simulink model "svpwmDCM"  (R2022b)
settings: Solver=VariableStepAuto  StartTime=0.0  StopTime=0.3  FixedStep=1e-5  RelTol=1e-4  EnableMultiTasking=on
libraries: spsIGBTDiodeLib x12, spsDiodeLib x6, spsSeriesRLCBranchLib x3, spsDCVoltageSourceLib x2, spsGroundLib x2, spsThreePhaseVIMeasurementLib x2, spsPermanentMagnetSynchronousMachineLib x1, spsAlphaBetaZerotodq0Lib x1, simulink x1, spsVoltageMeasurementLib x1, sps_lib x1
settings Model: Creator=Ranit  LastModifiedBy=ahmetcan.akuz
settings SolverCC: AlgebraicLoopSolver=TrustRegion
settings DataIOCC: ReturnWorkspaceOutputs=off
settings OptimizationCC: LifeSpan=inf
settings DebuggingCC: UnconnectedInputMsg=warning  UnconnectedOutputMsg=warning  UnconnectedLineMsg=warning  SFUnexpectedBacktrackingDiag=warning  SFNoUnconditionalDefaultTransitionDiag=warning  SFMachineParentedDataDiag=warning  ArithmeticOperatorsInVariantConditions=warning
settings ModelReferenceCC: EnableRefExpFcnMdlSchedulingChecks=on
settings SFSimCC: SimUseLocalCustomCode=off  CustomCodeUndefinedFunction=UseInterfaceOnly
settings RTWCC: RTWUseLocalCustomCode=off
settings CodeAppCC: StateflowObjectComments=on
settings GRTTargetCC: TargetLangStandard=C89/C90 (ANSI)
settings ConfigComp: CovMetricSettings=dw  CovSaveCumulativeToWorkspaceVar=on  CovSaveSingleToWorkspaceVar=on  CovExternalEMLEnable=off
settings SimscapeCC: SimscapeNormalizeSystem=off

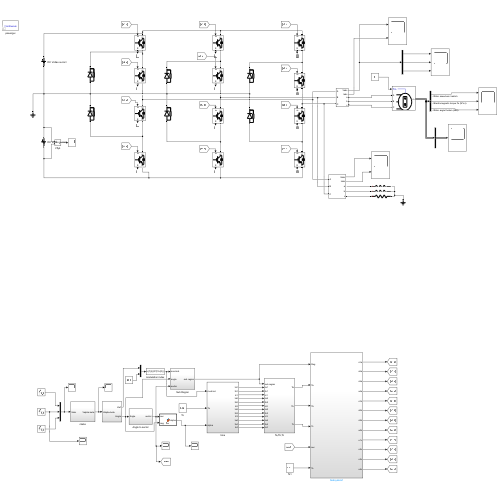
[thumbnail: Simulink's stored preview of the top-level diagram]
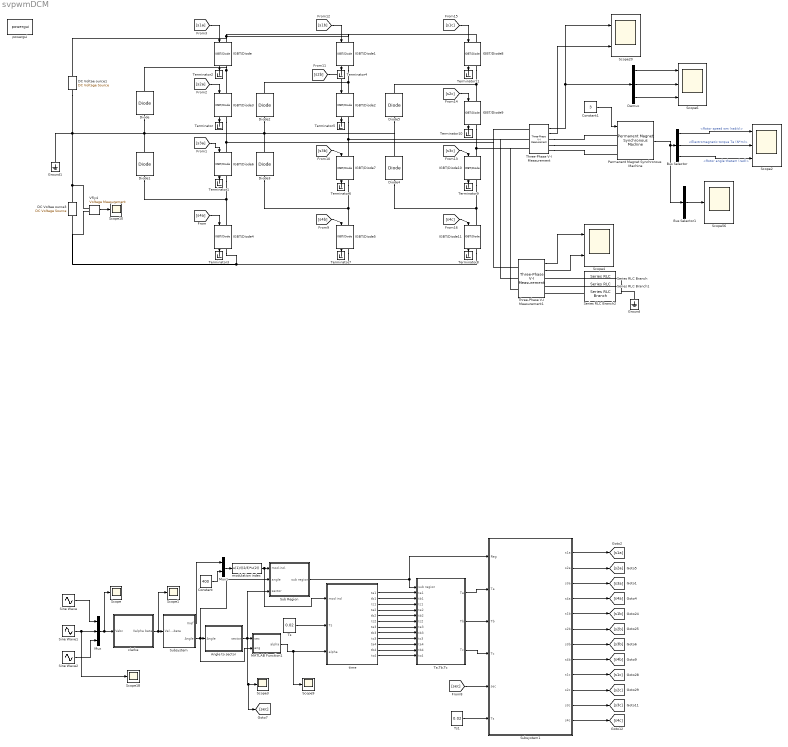
== system svpwmDCM ==
  Angle to sector : Subsystem
  Bus Selector : BusSelector  OutputSignals=Rotor speed wm (rad/s),Electromagnetic torque Te (N*m),Rotor angle thetam (rad)
  Bus Selector1 : BusSelector  OutputSignals=Stator current is_a (A),Stator current is_b (A),Stator current is_c (A)  OutputAsBus=on
  Constant : Constant  Value=400
  Constant1 : Constant  Value=3
  DC Voltae ource1 : spsDCVoltageSourceLib/DC Voltage Source  Amplitude=200  Measurements=None
  DC Voltae ource3 : spsDCVoltageSourceLib/DC Voltage Source  Amplitude=200  Measurements=None
  Demux : Demux  Outputs=3
  Diode{,1..5} (6 alike) : spsDiodeLib/Diode  Ron=0.001  Lon=0  Vf=0.8  IC=0  UseSnubber=off  Rs=500  Cs=250e-9  Measurements=off
  Ground : spsGroundLib/Ground  LConnTagsString=a
  Ground1 : spsGroundLib/Ground  LConnTagsString=a
  IGBT/Diode{,1..11} (12 alike) : spsIGBTDiodeLib/IGBT//Diode  Ron=1e-3  Rs=1e5  Cs=inf  Measurements=on
  MATLAB Function1 : MATLAB Function  TreatAsAtomicUnit=on
  Mux : Mux  Inputs=3
  Mux1 : Mux  Inputs=2
  Permanent Magnet Synchronous Machine : spsPermanentMagnetSynchronousMachineLib/Permanent Magnet Synchronous Machine  NbPhases=3  FluxDistribution=Sinusoidal  RotorType=Round  MechanicalLoad=Torque Tm  PresetModel=No  ShowDetailedParameters=on  MeasurementBus=off  Resistance=12.8  Inductance=8.5e-3  dqInductances=[0.002547 0.002816]  La=0.002682  MachineConstant=Flux linkage established by magnets (V.s)  Flux=0.22  VoltageCst=79.8072  TorqueCst=0.66  Flat=120  Mechanical=[2.26e-05 1.349e-05 2 0]  PolePairs=2  InitialConditions=[0,0, 0,0]  InitialConditions5ph=[0 0 0 0 0 0]  RefAngle=90 degrees behind phase A axis (modified Park)  IterativeDiscreteModel=Trapezoidal non iterative  TsBlock=-1  TsPowergui=0
  Scope{,1,3,9..10,18,56} (7 alike) : Scope
  Scope2 : Scope  NumInputPorts=3
  Scope20 : Scope  NumInputPorts=2
  Scope4 : Scope  NumInputPorts=2
  Scope6 : Scope  NumInputPorts=3
  Series RLC Branch : spsSeriesRLCBranchLib/Series RLC Branch  LConnTagsString=__new0  RConnTagsString=__new0  BranchType=R  Resistance=5  Inductance=20e-6  SetiL0=off  InitialCurrent=0  Capacitance=1e-6  Setx0=off  InitialVoltage=0  Measurements=None
  Series RLC Branch1 : spsSeriesRLCBranchLib/Series RLC Branch  LConnTagsString=__new0  RConnTagsString=__new0  BranchType=R  Resistance=5  Inductance=20e-6  SetiL0=off  InitialCurrent=0  Capacitance=1e-6  Setx0=off  InitialVoltage=0  Measurements=None
  Series RLC Branch2 : spsSeriesRLCBranchLib/Series RLC Branch  LConnTagsString=__new0  RConnTagsString=__new0  BranchType=R  Resistance=5  Inductance=20e-6  SetiL0=off  InitialCurrent=0  Capacitance=1e-6  Setx0=off  InitialVoltage=0  Measurements=None
  Sine Wave : Sin  Amplitude=230  Frequency=2*pi*50  SampleTime=0
  Sine Wave1 : Sin  Amplitude=230  Frequency=2*pi*50  Phase=4*pi/3  SampleTime=0
  Sine Wave2 : Sin  Amplitude=230  Frequency=2*pi*50  Phase=2*pi/3  SampleTime=0
  Sub Region : Subsystem
  Subsystem : Subsystem
  Subsystem1 : Subsystem
  Ta,Tb,Tc : Subsystem
  Terminator{,1..11} (12 alike) : Terminator
  Three-Phase V-I Measurement : spsThreePhaseVIMeasurementLib/Three-Phase V-I Measurement  VoltageMeasurement=phase-to-phase  SetLabelV=off  LabelV=Vabc  Vpu=off  VpuLL=off  CurrentMeasurement=yes  SetLabelI=off  LabelI=Iabc  Ipu=off  Pbase=100e6  Vbase=500e3  OutputType=Complex  PhasorSimulation=off  PSBequivalent=0
  Three-Phase V-I Measurement1 : spsThreePhaseVIMeasurementLib/Three-Phase V-I Measurement  VoltageMeasurement=phase-to-ground  SetLabelV=off  LabelV=Vabc  Vpu=off  VpuLL=off  CurrentMeasurement=yes  SetLabelI=off  LabelI=Iabc  Ipu=off  Pbase=100e6  Vbase=500e3  OutputType=Complex  PhasorSimulation=off  PSBequivalent=0
  Ts : Constant  Value=0.02
  Ts1 : Constant  Value=0.02
  Vfly4 : spsVoltageMeasurementLib/Voltage Measurement  PhasorSimulation=off  OutputType=Complex  PSBequivalent=0
  clarke : Subsystem
  modulation index : Fcn  Expr=u(1)/((2/3)*u(2))
  powergui : sps_lib/powergui  Priority=1  SimulationMode=Continuous  SampleTime=5e-4  frequency=60  Iterations=50  frequencyindice=0  Pbase=100e6  ErrMax=1e-4  UnitsV=kV  UnitsW=MW  buscounter=0  FunctionMessages=off  echomessages=off  EnableUseOfTLC=off  CurrentSourceSwitches=on  DisableSnubberDevices=off  DisableRonSwitches=off  DisableVfSwitches=off  DisplayEquations=off  AutomaticDiscreteSolvers=off  SolverType=Tustin/Backward Euler (TBE)  Interpol=off  ExternalGateDelay=off  methode=off  Ts=10  x0status=blocks  SPID=off  SwTol=0  HookPort=off  NonlinearTolerance=1e-4  nMaxIteration=100  ContinueOnMaxIteration=off  RestoreLinks=warning  ResistiveCurrentMeasurement=off  Frange=[0:2:500]  Ylog=off  Xlog=on  ShowGrid=off  save=off  variable=ZData  structure=ScopeData2  ZoomFFT=off  StartTime=0.0  cycles=1  DisplayStyle=1  fundamental=50  FreqAxis=off  MaxFrequency=1000  frequencyindicesteady=1  RmsSteady=1  display=off
  time : Subsystem
  wires:
  Sine Wave/1 -> Mux/1
  Sine Wave1/1 -> Scope18/1, Mux/2
  Sine Wave2/1 -> Mux/3
  Mux/1 -> clarke/1(Vabc), Scope/1
  clarke/1(Valpha beta) -> Scope1/1, Subsystem/1(Valpha-beta)
  Subsystem/1(Vref) -> Mux1/1
  Constant/1 -> Mux1/2
  Mux1/1 -> modulation index/1
  [s4a] -> IGBT/Diode4/1
  [s3a] -> IGBT/Diode6/1
  [s1a] -> IGBT/Diode/1
  [s2a] -> IGBT/Diode3/1
  Ts/1 -> time/2(Ts)
  time/1(ta1) -> Ta,Tb,Tc/2(ta1)
  time/2(tb1) -> Ta,Tb,Tc/3(tb1)
  time/3(tc1) -> Ta,Tb,Tc/4(tc1)
  time/4(ta2) -> Ta,Tb,Tc/5(ta2)
  time/5(tb2) -> Ta,Tb,Tc/6(tb2)
  time/6(tc2) -> Ta,Tb,Tc/7(tc2)
  time/7(ta3) -> Ta,Tb,Tc/8(ta3)
  time/9(tc3) -> Ta,Tb,Tc/10(tc3)
  time/10(ta4) -> Ta,Tb,Tc/11(ta4)
  time/11(tb4) -> Ta,Tb,Tc/12(tb4)
  time/12(tc4) -> Ta,Tb,Tc/13(tc4)
  time/8(tb3) -> Ta,Tb,Tc/9(tb3)
  modulation index/1 -> time/1(mod ind), Sub Region/1(mod.ind.)
  Subsystem/2(Angle) -> MATLAB Function1/2(ang), Sub Region/2(angle), Angle to sector/1(Angle)
  MATLAB Function1/1(alpha) -> Scope9/1, time/3(alpha)
  [s4b] -> IGBT/Diode5/1
  [s3b] -> IGBT/Diode7/1
  [s1b] -> IGBT/Diode1/1
  [s2b] -> IGBT/Diode2/1
  [s4c] -> IGBT/Diode11/1
  [s3c] -> IGBT/Diode10/1
  [s1c] -> IGBT/Diode8/1
  [s2c] -> IGBT/Diode9/1
  Vfly4/1 -> Scope10/1
  Sub Region/1(sub region) -> Subsystem1/1(Reg), Ta,Tb,Tc/1(sub region)
  Angle to sector/1(sector) -> Sub Region/3(sector), [sec], Scope3/1, MATLAB Function1/1(sec)
  Ta,Tb,Tc/1(Ta) -> Subsystem1/2(Ta)
  Ta,Tb,Tc/2(Tb) -> Subsystem1/3(Tb)
  Ta,Tb,Tc/3(Tc) -> Subsystem1/4(Tc)
  Subsystem1/1(s1a) -> [s1a]
  Subsystem1/2(s2a) -> [s2a]
  Subsystem1/3(s3a) -> [s3a]
  Subsystem1/4(s4a) -> [s4a]
  Subsystem1/6(s2b) -> [s2b]
  Subsystem1/5(s1b) -> [s1b]
  Subsystem1/7(s3b) -> [s3b]
  Subsystem1/8(s4b) -> [s4b]
  Subsystem1/9(s1c) -> [s1c]
  Subsystem1/10(s2c) -> [s2c]
  Subsystem1/11(s3c) -> [s3c]
  Subsystem1/12(s4c) -> [s4c]
  [sec] -> Subsystem1/5(sec)
  Ts1/1 -> Subsystem1/6(Ts)
  Permanent Magnet Synchronous Machine/1 -> Bus Selector1/1, Bus Selector/1
  Constant1/1 -> Permanent Magnet Synchronous Machine/1
  Bus Selector/1 -> Scope2/1  "<Rotor speed wm (rad/s)>"
  Bus Selector/2 -> Scope2/2  "<Electromagnetic torque Te (N*m)>"
  Bus Selector/3 -> Scope2/3  "<Rotor angle thetam (rad)>"
  Bus Selector1/1 -> Scope56/1
  IGBT/Diode3/1 -> Terminator/1
  IGBT/Diode6/1 -> Terminator1/1
  IGBT/Diode/1 -> Terminator2/1
  IGBT/Diode4/1 -> Terminator3/1
  IGBT/Diode1/1 -> Terminator4/1
  IGBT/Diode2/1 -> Terminator5/1
  IGBT/Diode7/1 -> Terminator6/1
  IGBT/Diode5/1 -> Terminator7/1
  IGBT/Diode11/1 -> Terminator8/1
  IGBT/Diode10/1 -> Terminator9/1
  IGBT/Diode9/1 -> Terminator10/1
  IGBT/Diode8/1 -> Terminator11/1
  Three-Phase V-I Measurement/2 -> Scope20/2
  Three-Phase V-I Measurement1/1 -> Scope4/1
  Three-Phase V-I Measurement1/2 -> Scope4/2
  Demux/1 -> Scope6/1
  Demux/2 -> Scope6/2
  Demux/3 -> Scope6/3
  Three-Phase V-I Measurement/1 -> Demux/1, Scope20/1
  connections:
  Diode1/LConn1 -- IGBT/Diode4/LConn1 -- IGBT/Diode6/RConn1
  Diode/RConn1 -- IGBT/Diode3/LConn1 -- IGBT/Diode/RConn1
  IGBT/Diode8/LConn1 -- IGBT/Diode1/LConn1 -- IGBT/Diode/LConn1 -- DC Voltae ource1/RConn1
  IGBT/Diode5/RConn1 -- IGBT/Diode11/RConn1 -- IGBT/Diode4/RConn1 -- DC Voltae ource3/LConn1 -- Vfly4/LConn2
  Vfly4/LConn1 -- DC Voltae ource3/RConn1 -- DC Voltae ource1/LConn1 -- Diode/LConn1 -- Diode2/LConn1 -- Diode4/RConn1 -- Diode5/LConn1 -- Diode3/RConn1 -- Diode1/RConn1 -- Ground1/LConn1
  Diode3/LConn1 -- IGBT/Diode7/RConn1 -- IGBT/Diode5/LConn1
  Diode2/RConn1 -- IGBT/Diode2/LConn1 -- IGBT/Diode1/RConn1
  Diode4/LConn1 -- IGBT/Diode11/LConn1 -- IGBT/Diode10/RConn1
  Diode5/RConn1 -- IGBT/Diode9/LConn1 -- IGBT/Diode8/RConn1
  Three-Phase V-I Measurement/LConn3 -- Three-Phase V-I Measurement1/LConn3 -- IGBT/Diode10/LConn1 -- IGBT/Diode9/RConn1
  Three-Phase V-I Measurement/LConn1 -- Three-Phase V-I Measurement1/LConn1 -- IGBT/Diode6/LConn1 -- IGBT/Diode3/RConn1
  Three-Phase V-I Measurement1/LConn2 -- Three-Phase V-I Measurement/LConn2 -- IGBT/Diode7/LConn1 -- IGBT/Diode2/RConn1
  Three-Phase V-I Measurement/RConn1 -- Permanent Magnet Synchronous Machine/LConn1
  Three-Phase V-I Measurement/RConn2 -- Permanent Magnet Synchronous Machine/LConn2
  Three-Phase V-I Measurement/RConn3 -- Permanent Magnet Synchronous Machine/LConn3
  Series RLC Branch2/LConn1 -- Three-Phase V-I Measurement1/RConn3
  Series RLC Branch1/LConn1 -- Three-Phase V-I Measurement1/RConn2
  Series RLC Branch/LConn1 -- Three-Phase V-I Measurement1/RConn1
  Series RLC Branch/RConn1 -- Ground/LConn1 -- Series RLC Branch2/RConn1 -- Series RLC Branch1/RConn1

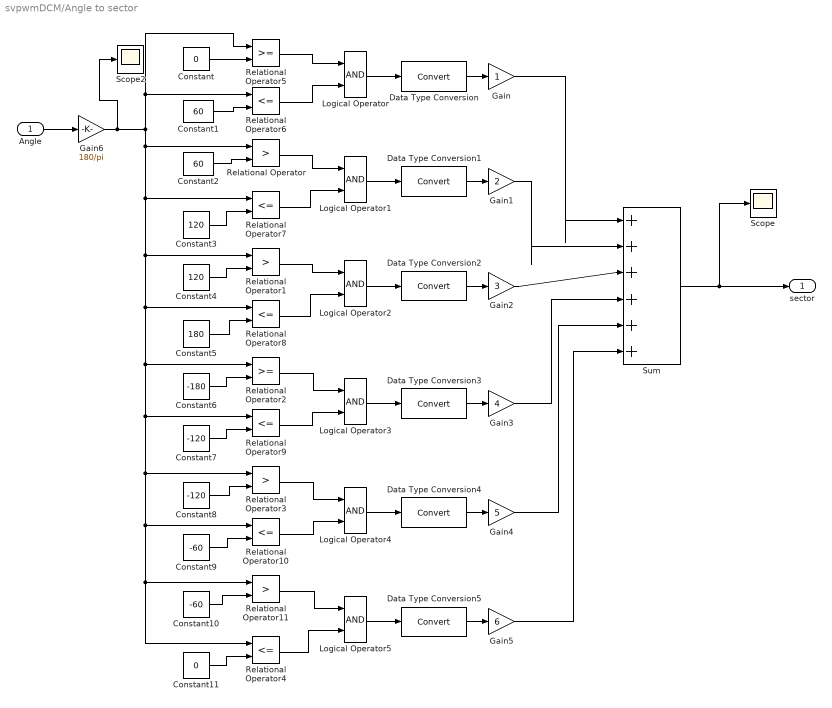
== system svpwmDCM/Angle to sector ==
  Angle : Inport
  Constant : Constant  Value=0
  Constant1 : Constant  Value=60
  Constant10 : Constant  Value=-60
  Constant11 : Constant  Value=0
  Constant2 : Constant  Value=60
  Constant3 : Constant  Value=120
  Constant4 : Constant  Value=120
  Constant5 : Constant  Value=180
  Constant6 : Constant  Value=-180
  Constant7 : Constant  Value=-120
  Constant8 : Constant  Value=-120
  Constant9 : Constant  Value=-60
  Data Type Conversion{,1..5} (6 alike) : DataTypeConversion  SaturateOnIntegerOverflow=off  RndMeth=Floor
  Gain : Gain
  Gain1 : Gain  Gain=2
  Gain2 : Gain  Gain=3
  Gain3 : Gain  Gain=4
  Gain4 : Gain  Gain=5
  Gain5 : Gain  Gain=6
  Gain6 : Gain  Gain=180/pi
  Logical Operator{,1..5} (6 alike) : Logic  AllPortsSameDT=off  OutDataTypeStr=boolean
  Relational Operator{,1,3,11} (4 alike) : RelationalOperator  Operator=>  OutDataTypeStr=boolean  InputSameDT=off
  Relational Operator{4,6..10} (6 alike) : RelationalOperator  Operator=<=  OutDataTypeStr=boolean  InputSameDT=off
  Relational Operator2 : RelationalOperator  OutDataTypeStr=boolean  InputSameDT=off
  Relational Operator5 : RelationalOperator  OutDataTypeStr=boolean  InputSameDT=off
  Scope : Scope
  Scope2 : Scope
  Sum : Sum  Inputs=|++++++
  sector : Outport
  wires:
  Constant/1 -> Relational Operator5/2
  Constant1/1 -> Relational Operator6/2
  Constant2/1 -> Relational Operator/2
  Constant3/1 -> Relational Operator7/2
  Gain6/1 -> Scope2/1, Relational Operator5/1, Relational Operator6/1, Relational Operator4/1, Relational Operator11/1, Relational Operator10/1, Relational Operator3/1, Relational Operator9/1, Relational Operator2/1, Relational Operator8/1, Relational Operator1/1, Relational Operator7/1, Relational Operator/1
  Constant5/1 -> Relational Operator8/2
  Constant6/1 -> Relational Operator2/2
  Constant7/1 -> Relational Operator9/2
  Constant8/1 -> Relational Operator3/2
  Constant9/1 -> Relational Operator10/2
  Constant10/1 -> Relational Operator11/2
  Constant11/1 -> Relational Operator4/2
  Constant4/1 -> Relational Operator1/2
  Relational Operator11/1 -> Logical Operator5/1
  Relational Operator4/1 -> Logical Operator5/2
  Relational Operator3/1 -> Logical Operator4/1
  Relational Operator10/1 -> Logical Operator4/2
  Relational Operator2/1 -> Logical Operator3/1
  Relational Operator9/1 -> Logical Operator3/2
  Relational Operator5/1 -> Logical Operator/1
  Relational Operator6/1 -> Logical Operator/2
  Relational Operator/1 -> Logical Operator1/1
  Relational Operator7/1 -> Logical Operator1/2
  Relational Operator1/1 -> Logical Operator2/1
  Relational Operator8/1 -> Logical Operator2/2
  Gain4/1 -> Sum/5
  Gain3/1 -> Sum/4
  Gain5/1 -> Sum/6
  Gain2/1 -> Sum/3
  Gain1/1 -> Sum/2
  Gain/1 -> Sum/1
  Sum/1 -> Scope/1, sector/1
  Angle/1 -> Gain6/1
  Logical Operator/1 -> Data Type Conversion/1
  Data Type Conversion/1 -> Gain/1
  Data Type Conversion1/1 -> Gain1/1
  Logical Operator1/1 -> Data Type Conversion1/1
  Data Type Conversion2/1 -> Gain2/1
  Logical Operator2/1 -> Data Type Conversion2/1
  Data Type Conversion3/1 -> Gain3/1
  Logical Operator3/1 -> Data Type Conversion3/1
  Data Type Conversion4/1 -> Gain4/1
  Logical Operator4/1 -> Data Type Conversion4/1
  Data Type Conversion5/1 -> Gain5/1
  Logical Operator5/1 -> Data Type Conversion5/1

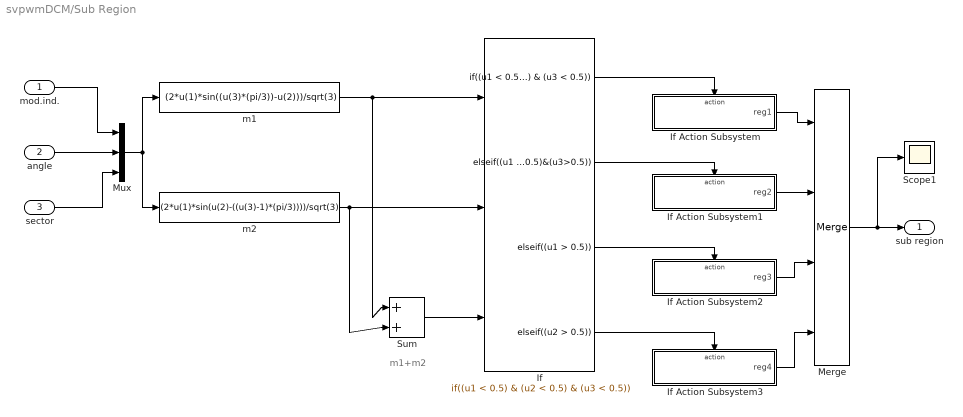
== system svpwmDCM/Sub Region ==
  note: m1+m2
  mod.ind. : Inport
  angle : Inport  Port=2
  sector : Inport  Port=3
  If : If  NumInputs=3  IfExpression=(u1 < 0.5) & (u2 < 0.5) & (u3 < 0.5)  ElseIfExpressions=(u1 < 0.5)&(u2 < 0.5)&(u3>0.5),(u1 > 0.5),(u2 > 0.5)  ShowElse=off
  If Action Subsystem : Subsystem  TreatAsAtomicUnit=on
  If Action Subsystem1 : Subsystem  TreatAsAtomicUnit=on
  If Action Subsystem2 : Subsystem  TreatAsAtomicUnit=on
  If Action Subsystem3 : Subsystem  TreatAsAtomicUnit=on
  Merge : Merge  Inputs=4
  Mux : Mux  Inputs=3
  Scope1 : Scope
  Sum : Sum  Inputs=|++
  m1 : Fcn  Expr=(2*u(1)*sin((u(3)*(pi/3))-u(2)))/sqrt(3)
  m2 : Fcn  Expr=(2*u(1)*sin(u(2)-((u(3)-1)*(pi/3))))/sqrt(3)
  sub region : Outport
  wires:
  mod.ind./1 -> Mux/1
  angle/1 -> Mux/2
  sector/1 -> Mux/3
  Mux/1 -> m1/1, m2/1
  m1/1 -> Sum/1, If/1
  m2/1 -> If/2, Sum/2
  Sum/1 -> If/3
  If/1 -> If Action Subsystem/Action
  If Action Subsystem/1(reg1) -> Merge/1
  If Action Subsystem3/1(reg4) -> Merge/4
  If Action Subsystem2/1(reg3) -> Merge/3
  If Action Subsystem1/1(reg2) -> Merge/2
  Merge/1 -> sub region/1, Scope1/1
  If/2 -> If Action Subsystem1/Action
  If/3 -> If Action Subsystem2/Action
  If/4 -> If Action Subsystem3/Action

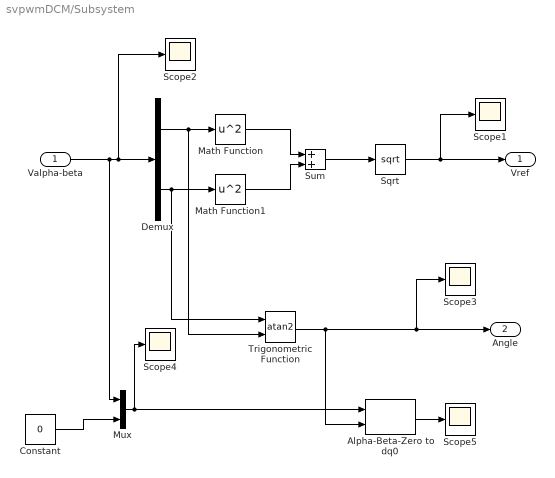
== system svpwmDCM/Subsystem ==
  Valpha-beta : Inport
  Alpha-Beta-Zero to dq0 : spsAlphaBetaZerotodq0Lib/Alpha-Beta-Zero to dq0  Alignment=90 degrees behind phase A axis
  Constant : Constant  Value=0
  Demux : Demux  Outputs=2
  Math Function : Math  Operator=square  SignedPower=on
  Math Function1 : Math  Operator=square  SignedPower=on
  Mux : Mux  Inputs=2
  Scope{1..5} (5 alike) : Scope
  Sqrt : Sqrt
  Sum : Sum  Inputs=|++
  Trigonometric Function : Trigonometry  Operator=atan2
  Vref : Outport
  Angle : Outport  Port=2
  wires:
  Valpha-beta/1 -> Mux/1, Scope2/1, Demux/1
  Demux/1 -> Trigonometric Function/2, Math Function/1
  Demux/2 -> Trigonometric Function/1, Math Function1/1
  Math Function/1 -> Sum/1
  Math Function1/1 -> Sum/2
  Sum/1 -> Sqrt/1
  Sqrt/1 -> Vref/1, Scope1/1
  Trigonometric Function/1 -> Alpha-Beta-Zero to dq0/2, Angle/1, Scope3/1
  Constant/1 -> Mux/2
  Mux/1 -> Scope4/1, Alpha-Beta-Zero to dq0/1
  Alpha-Beta-Zero to dq0/1 -> Scope5/1

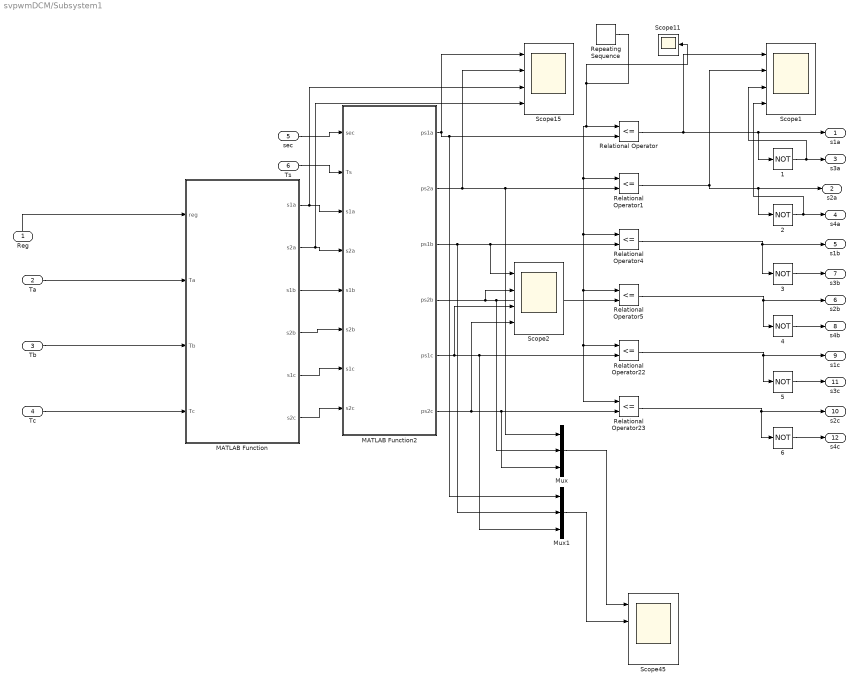
== system svpwmDCM/Subsystem1 ==
  Reg : Inport
  Ta : Inport  Port=2
  Tb : Inport  Port=3
  Tc : Inport  Port=4
  sec : Inport  Port=5
  Ts : Inport  Port=6
  {1..6} (6 alike) : Logic  Operator=NOT  AllPortsSameDT=off  OutDataTypeStr=boolean
  MATLAB Function : MATLAB Function  TreatAsAtomicUnit=on
  MATLAB Function2 : MATLAB Function  TreatAsAtomicUnit=on
  Mux : Mux  Inputs=3
  Mux1 : Mux  Inputs=3
  Relational Operator{,1,4..5,22..23} (6 alike) : RelationalOperator  Operator=<=  OutDataTypeStr=boolean  InputSameDT=off
  Repeating Sequence : simulink/Sources/Repeating Sequence  rep_seq_t=[0 1 2]*[1/6000]  rep_seq_y=[0 0.01 0]
  Scope{1..2,15,45} (4 alike) : Scope  NumInputPorts=4
  Scope11 : Scope
  s1a : Outport
  s2a : Outport  Port=2
  s3a : Outport  Port=3
  s4a : Outport  Port=4
  s1b : Outport  Port=5
  s2b : Outport  Port=6
  s3b : Outport  Port=7
  s4b : Outport  Port=8
  s1c : Outport  Port=9
  s2c : Outport  Port=10
  s3c : Outport  Port=11
  s4c : Outport  Port=12
  wires:
  Reg/1 -> MATLAB Function/1(reg)
  MATLAB Function2/3(ps1b) -> Mux1/2, Scope2/1, Relational Operator4/2
  MATLAB Function2/4(ps2b) -> Scope2/2, Mux/2, Relational Operator5/2
  MATLAB Function2/2(ps2a) -> Relational Operator1/2, Mux/1, Scope15/2
  Relational Operator4/1 -> s1b/1, 3/1
  MATLAB Function2/6(ps2c) -> Scope2/4, Mux/3, Relational Operator23/2
  Relational Operator5/1 -> s2b/1, 4/1
  Repeating Sequence/1 -> Relational Operator/1, Relational Operator23/1, Relational Operator22/1, Relational Operator5/1, Relational Operator4/1, Relational Operator1/1, Scope11/1
  Relational Operator22/1 -> s1c/1, 5/1
  Relational Operator23/1 -> s2c/1, 6/1
  MATLAB Function/5(s1c) -> MATLAB Function2/7(s1c)
  MATLAB Function/6(s2c) -> MATLAB Function2/8(s2c)
  MATLAB Function/4(s2b) -> MATLAB Function2/6(s2b)
  Tb/1 -> MATLAB Function/3(Tb)
  Tc/1 -> MATLAB Function/4(Tc)
  Ta/1 -> MATLAB Function/2(Ta)
  MATLAB Function2/1(ps1a) -> Mux1/1, Relational Operator/2, Scope15/1
  4/1 -> s4b/1
  MATLAB Function/1(s1a) -> Scope15/3, MATLAB Function2/3(s1a)
  MATLAB Function/2(s2a) -> Scope15/4, MATLAB Function2/4(s2a)
  Relational Operator1/1 -> s2a/1, 2/1, Scope1/2
  2/1 -> Scope1/4, s4a/1
  6/1 -> s4c/1
  MATLAB Function/3(s1b) -> MATLAB Function2/5(s1b)
  1/1 -> Scope1/3, s3a/1
  3/1 -> s3b/1
  5/1 -> s3c/1
  sec/1 -> MATLAB Function2/1(sec)
  Ts/1 -> MATLAB Function2/2(Ts)
  Relational Operator/1 -> Scope1/1, s1a/1, 1/1
  MATLAB Function2/5(ps1c) -> Scope2/3, Mux1/3, Relational Operator22/2
  Mux/1 -> Scope45/1
  Mux1/1 -> Scope45/2

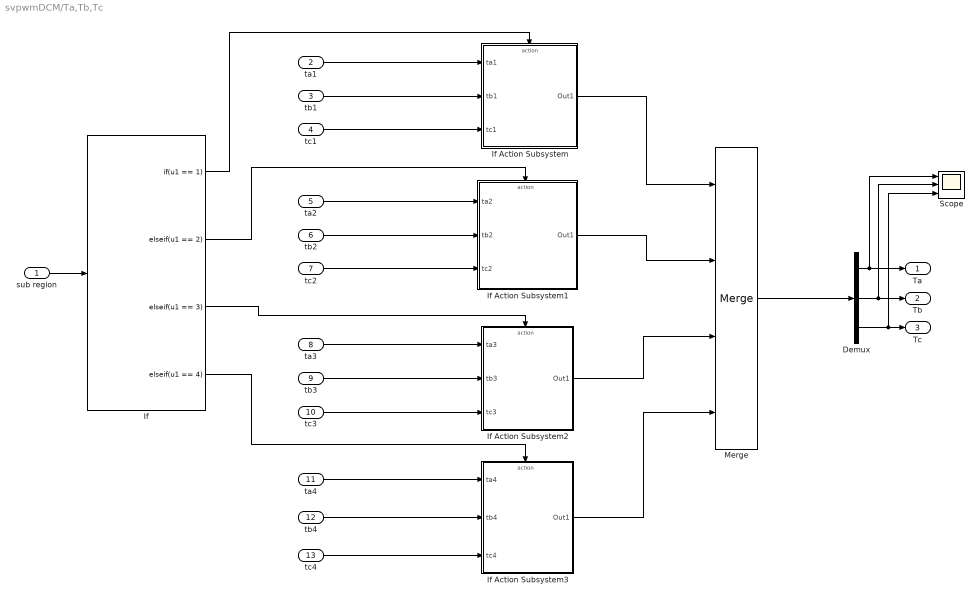
== system svpwmDCM/Ta,Tb,Tc ==
  sub region : Inport
  ta1 : Inport  Port=2
  tb1 : Inport  Port=3
  tc1 : Inport  Port=4
  ta2 : Inport  Port=5
  tb2 : Inport  Port=6
  tc2 : Inport  Port=7
  ta3 : Inport  Port=8
  tb3 : Inport  Port=9
  tc3 : Inport  Port=10
  ta4 : Inport  Port=11
  tb4 : Inport  Port=12
  tc4 : Inport  Port=13
  Demux : Demux  Outputs=3
  If : If  IfExpression=u1 == 1  ElseIfExpressions=u1 == 2,u1 == 3,u1 == 4  ShowElse=off  ZeroCross=off
  If Action Subsystem : Subsystem  TreatAsAtomicUnit=on
  If Action Subsystem1 : Subsystem  TreatAsAtomicUnit=on
  If Action Subsystem2 : Subsystem  TreatAsAtomicUnit=on
  If Action Subsystem3 : Subsystem  TreatAsAtomicUnit=on
  Merge : Merge  Inputs=4
  Scope : Scope  NumInputPorts=3
  Ta : Outport
  Tb : Outport  Port=2
  Tc : Outport  Port=3
  wires:
  sub region/1 -> If/1
  If/1 -> If Action Subsystem/Action
  If/2 -> If Action Subsystem1/Action
  tb3/1 -> If Action Subsystem2/2(tb3)
  ta3/1 -> If Action Subsystem2/1(ta3)
  tc3/1 -> If Action Subsystem2/3(tc3)
  tb2/1 -> If Action Subsystem1/2(tb2)
  ta2/1 -> If Action Subsystem1/1(ta2)
  tc2/1 -> If Action Subsystem1/3(tc2)
  tc1/1 -> If Action Subsystem/3(tc1)
  tb1/1 -> If Action Subsystem/2(tb1)
  ta1/1 -> If Action Subsystem/1(ta1)
  ta4/1 -> If Action Subsystem3/1(ta4)
  tb4/1 -> If Action Subsystem3/2(tb4)
  tc4/1 -> If Action Subsystem3/3(tc4)
  If Action Subsystem1/1(Out1) -> Merge/2
  If Action Subsystem2/1(Out1) -> Merge/3
  If Action Subsystem/1(Out1) -> Merge/1
  If Action Subsystem3/1(Out1) -> Merge/4
  Merge/1 -> Demux/1
  Demux/1 -> Scope/1, Ta/1
  Demux/2 -> Tb/1, Scope/2
  Demux/3 -> Scope/3, Tc/1
  If/3 -> If Action Subsystem2/Action
  If/4 -> If Action Subsystem3/Action

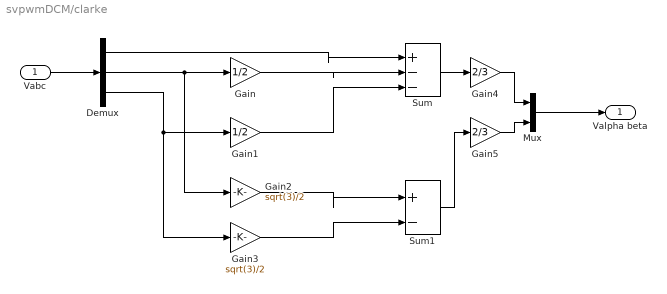
== system svpwmDCM/clarke ==
  Vabc : Inport
  Demux : Demux  Outputs=3
  Gain : Gain  Gain=1/2
  Gain1 : Gain  Gain=1/2
  Gain2 : Gain  Gain=sqrt(3)/2
  Gain3 : Gain  Gain=sqrt(3)/2
  Gain4 : Gain  Gain=2/3
  Gain5 : Gain  Gain=2/3
  Mux : Mux  Inputs=2
  Sum : Sum  Inputs=|+--
  Sum1 : Sum  Inputs=|+-
  Valpha beta : Outport
  wires:
  Vabc/1 -> Demux/1
  Demux/1 -> Sum/1
  Demux/2 -> Gain2/1, Gain/1
  Gain/1 -> Sum/2
  Demux/3 -> Gain1/1, Gain3/1
  Gain1/1 -> Sum/3
  Gain2/1 -> Sum1/1
  Gain3/1 -> Sum1/2
  Mux/1 -> Valpha beta/1
  Sum/1 -> Gain4/1
  Gain4/1 -> Mux/1
  Sum1/1 -> Gain5/1
  Gain5/1 -> Mux/2

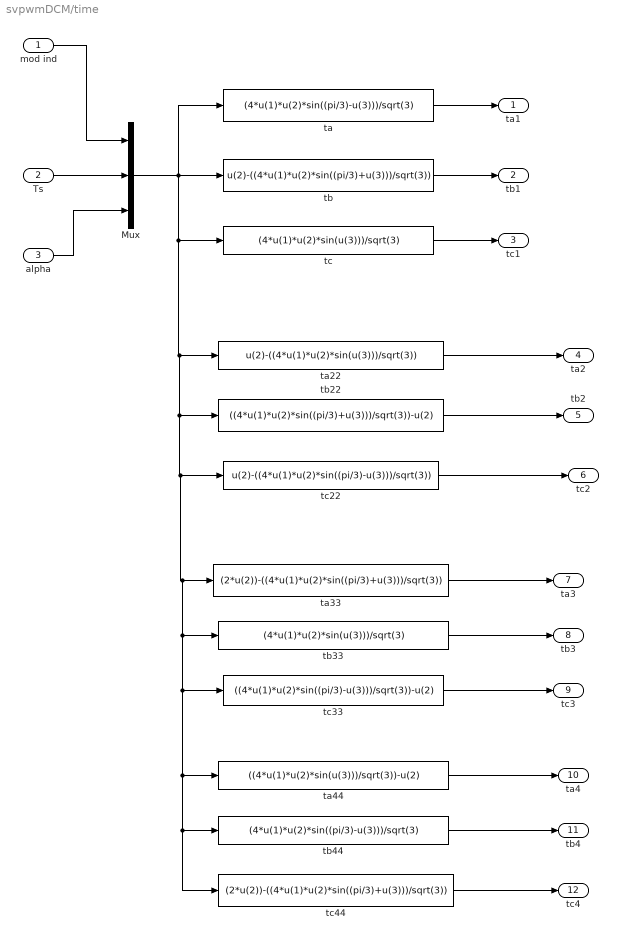
== system svpwmDCM/time ==
  mod ind : Inport
  Ts : Inport  Port=2
  alpha : Inport  Port=3
  Mux : Mux  Inputs=3
  ta : Fcn  Expr=(4*u(1)*u(2)*sin((pi/3)-u(3)))/sqrt(3)
  ta22 : Fcn  Expr=u(2)-((4*u(1)*u(2)*sin(u(3)))/sqrt(3))
  ta33 : Fcn  Expr=(2*u(2))-((4*u(1)*u(2)*sin((pi/3)+u(3)))/sqrt(3))
  ta44 : Fcn  Expr=((4*u(1)*u(2)*sin(u(3)))/sqrt(3))-u(2)
  tb : Fcn  Expr=u(2)-((4*u(1)*u(2)*sin((pi/3)+u(3)))/sqrt(3))
  tb22 : Fcn  Expr=((4*u(1)*u(2)*sin((pi/3)+u(3)))/sqrt(3))-u(2)
  tb33 : Fcn  Expr=(4*u(1)*u(2)*sin(u(3)))/sqrt(3)
  tb44 : Fcn  Expr=(4*u(1)*u(2)*sin((pi/3)-u(3)))/sqrt(3)
  tc : Fcn  Expr=(4*u(1)*u(2)*sin(u(3)))/sqrt(3)
  tc22 : Fcn  Expr=u(2)-((4*u(1)*u(2)*sin((pi/3)-u(3)))/sqrt(3))
  tc33 : Fcn  Expr=((4*u(1)*u(2)*sin((pi/3)-u(3)))/sqrt(3))-u(2)
  tc44 : Fcn  Expr=(2*u(2))-((4*u(1)*u(2)*sin((pi/3)+u(3)))/sqrt(3))
  ta1 : Outport
  tb1 : Outport  Port=2
  tc1 : Outport  Port=3
  ta2 : Outport  Port=4
  tb2 : Outport  Port=5
  tc2 : Outport  Port=6
  ta3 : Outport  Port=7
  tb3 : Outport  Port=8
  tc3 : Outport  Port=9
  ta4 : Outport  Port=10
  tb4 : Outport  Port=11
  tc4 : Outport  Port=12
  wires:
  mod ind/1 -> Mux/1
  Ts/1 -> Mux/2
  alpha/1 -> Mux/3
  ta/1 -> ta1/1
  tb/1 -> tb1/1
  tc/1 -> tc1/1
  ta22/1 -> ta2/1
  tb22/1 -> tb2/1
  tc22/1 -> tc2/1
  ta33/1 -> ta3/1
  tc33/1 -> tc3/1
  tb33/1 -> tb3/1
  Mux/1 -> tc/1, ta22/1, tb33/1, tb44/1, tc44/1, ta44/1, tc33/1, ta33/1, tc22/1, tb22/1, tb/1, ta/1
  ta44/1 -> ta4/1
  tb44/1 -> tb4/1
  tc44/1 -> tc4/1

== system svpwmDCM/Sub Region/If Action Subsystem ==
  Action Port : ActionPort  ActionPortLabel=if((u1 < 0.5) & (u2 < 0.5) & (u3 < 0.5))
  Constant : Constant
  reg1 : Outport
  wires:
  Constant/1 -> reg1/1

== system svpwmDCM/Sub Region/If Action Subsystem1 ==
  Action Port : ActionPort  ActionPortLabel=elseif((u1 < 0.5)&(u2 < 0.5)&(u3>0.5))
  Constant : Constant  Value=2
  reg2 : Outport
  wires:
  Constant/1 -> reg2/1

== system svpwmDCM/Sub Region/If Action Subsystem2 ==
  Action Port : ActionPort  ActionPortLabel=elseif((u1 > 0.5))
  Constant : Constant  Value=3
  reg3 : Outport
  wires:
  Constant/1 -> reg3/1

== system svpwmDCM/Sub Region/If Action Subsystem3 ==
  Action Port : ActionPort  ActionPortLabel=elseif((u2 > 0.5))
  Constant : Constant  Value=4
  reg4 : Outport
  wires:
  Constant/1 -> reg4/1

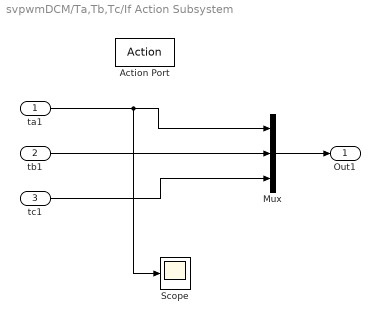
== system svpwmDCM/Ta,Tb,Tc/If Action Subsystem ==
  ta1 : Inport
  tb1 : Inport  Port=2
  tc1 : Inport  Port=3
  Action Port : ActionPort  ActionPortLabel=if(u1 == 1)
  Mux : Mux  Inputs=3
  Scope : Scope
  Out1 : Outport
  wires:
  ta1/1 -> Scope/1, Mux/1
  tb1/1 -> Mux/2
  tc1/1 -> Mux/3
  Mux/1 -> Out1/1

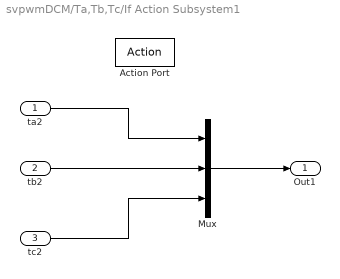
== system svpwmDCM/Ta,Tb,Tc/If Action Subsystem1 ==
  ta2 : Inport
  tb2 : Inport  Port=2
  tc2 : Inport  Port=3
  Action Port : ActionPort  ActionPortLabel=elseif(u1 == 2)
  Mux : Mux  Inputs=3
  Out1 : Outport
  wires:
  tb2/1 -> Mux/2
  ta2/1 -> Mux/1
  tc2/1 -> Mux/3
  Mux/1 -> Out1/1

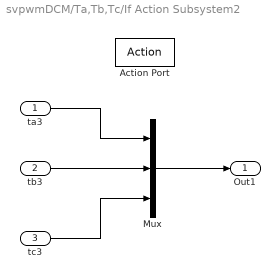
== system svpwmDCM/Ta,Tb,Tc/If Action Subsystem2 ==
  ta3 : Inport
  tb3 : Inport  Port=2
  tc3 : Inport  Port=3
  Action Port : ActionPort  ActionPortLabel=elseif(u1 == 3)
  Mux : Mux  Inputs=3
  Out1 : Outport
  wires:
  tb3/1 -> Mux/2
  ta3/1 -> Mux/1
  tc3/1 -> Mux/3
  Mux/1 -> Out1/1

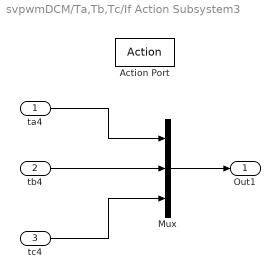
== system svpwmDCM/Ta,Tb,Tc/If Action Subsystem3 ==
  ta4 : Inport
  tb4 : Inport  Port=2
  tc4 : Inport  Port=3
  Action Port : ActionPort  ActionPortLabel=elseif(u1 == 4)
  Mux : Mux  Inputs=3
  Out1 : Outport
  wires:
  ta4/1 -> Mux/1
  tb4/1 -> Mux/2
  tc4/1 -> Mux/3
  Mux/1 -> Out1/1

== matlab function svpwmDCM/MATLAB Function1 ==
  data: sec input; alpha output; ang input
function alpha = fcn(sec,ang)
alpha=0;
if(sec==1)
  alpha=ang;
end
if(sec==2)
  alpha=ang-(pi/3);
end
if(sec==3)
  alpha=ang-(2*pi/3);
end
if(sec==4)
  alpha=pi+ang;
end
if(sec==5)
  alpha=(2*pi/3)+ang;
end
if(sec==6)
  alpha=(pi/3)+ang;
end

== matlab function svpwmDCM/Subsystem1/MATLAB Function ==
  data: reg input; s1a output; Ta input; Tb input; Tc input; s2a output; s1b output; s2b output; s1c output; s2c output
function [s1a,s2a,s1b,s2b,s1c,s2c] = fcn(reg,Ta,Tb,Tc)
s1a=0;
s2a=0;
s1b=0;
s2b=0;
s1c=0;
s2c=0;
if(reg==1)
    s1a=Ta/4+Tc/4+Tb/4;
    s2a=Ta/2+Tc/2+Tb/4+Tb/2;
    s1b=Tc/4+Tb/4;
    s2b=Tc/2+Ta/4+Tb/4+Tb/2;
    s1c=Tb/4;
    s2c=Tb/4+Tb/2+Ta/4+Tc/4;
end
if(reg==2)
    s1a=Tc/4+Ta/4+Tb/2;
    s2a=(Ta+Tb+Tc)/2;
    s1b=Tc/4;
    s2b=Tc/2+Tb/2+Ta/4;
    s1c=0;
    s2c=Ta/4+Tc/4;
end
if(reg==3)
    s1a=Tb/2+Tc/2+Ta/4;
    s2a=(Ta+Tb+Tc)/2;
    s1b=0;
    s2b=Tb/2+Ta/4;
    s1c=0;
    s2c=Ta/4;
end
if(reg==4)
    s1a=Tb/2+Ta/2+Tc/4;
    s2a=(Ta+Tb+Tc)/2;
    s1b=Ta/2++Tc/4;
    s2b=(Ta+Tb+Tc)/2;
    s1c=0;
    s2c=Tc/4;
end

== matlab function svpwmDCM/Subsystem1/MATLAB Function2 ==
  data: sec input; ps1a output; Ts input; s1a input; s2a input; s1b input; s2b input; s1c input; s2c input; ps2a output; ps1b output; ps2b output; ps1c output; ps2c output
function [ps1a,ps2a,ps1b,ps2b,ps1c,ps2c] = fcn(sec,Ts,s1a,s2a,s1b,s2b,s1c,s2c)
ps1a=0;
ps2a=0;
ps1b=0;
ps2b=0;
ps1c=0;
ps2c=0;
if(sec==1)
    ps1a=s1a;
    ps2a=s2a;
    ps1b=s1b;
    ps2b=s2b;
    ps1c=s1c;
    ps2c=s2c;
end
if(sec==2)
    ps1a=Ts/2-s2b;
    ps2a=Ts/2-s1b;
    ps1b=Ts/2-s2c;
    ps2b=Ts/2-s1c;
    ps1c=Ts/2-s2a;
    ps2c=Ts/2-s1a;
end
if(sec==3)
    ps1a=s1c;
    ps2a=s2c;
    ps1b=s1a;
    ps2b=s2a;
    ps1c=s1b;
    ps2c=s2b;
end
if(sec==4)
    ps1a=Ts/2-s2a;
    ps2a=Ts/2-s1a;
    ps1b=Ts/2-s2b;
    ps2b=Ts/2-s1b;
    ps1c=Ts/2-s2c;
    ps2c=Ts/2-s1c;
end
if(sec==5)
    ps1a=s1b;
    ps2a=s2b;
    ps1b=s1c;
    ps2b=s2c;
    ps1c=s1a;
    ps2c=s2a;
end
if(sec==6)
    ps1a=Ts/2-s2c;
    ps2a=Ts/2-s1c;
    ps1b=Ts/2-s2a;
    ps2b=Ts/2-s1a;
    ps1c=Ts/2-s2b;
    ps2c=Ts/2-s1b;
end
